simulink model "Sedimentation"  (R2024b)
settings: Solver=VariableStepAuto  StartTime=0.0  StopTime=1000  RelTol=1e-3
values from neighbouring files (symbols this model uses):
  b = Q_p/Q_in    (= 0.99)    [Input.m]
  D = Q_in/V    (= 0.166666666667)    [Input.m]
  f_ns = 1E-5    (= 1e-05)    [Input.m]
  h = 0.1    [Input.m]
  n = 5    [Input.m]
  r = Q_r/Q_in    (= 0.01)    [Input.m]
  r_h = 2E-6    (= 2e-06)    [Input.m]
  r_p = 1E-4    (= 0.0001)    [Input.m]
  v_0 = 10.42    [Input.m]
undefined symbols (not defined in the file or in its folder): X_in
settings Model: Creator=luima  LastModifiedBy=luima

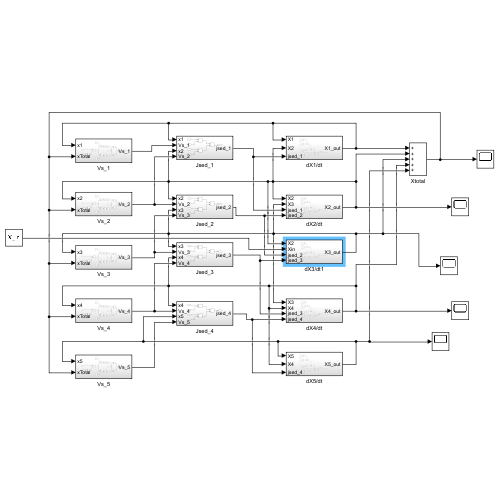
[thumbnail: Simulink's stored preview of the top-level diagram]
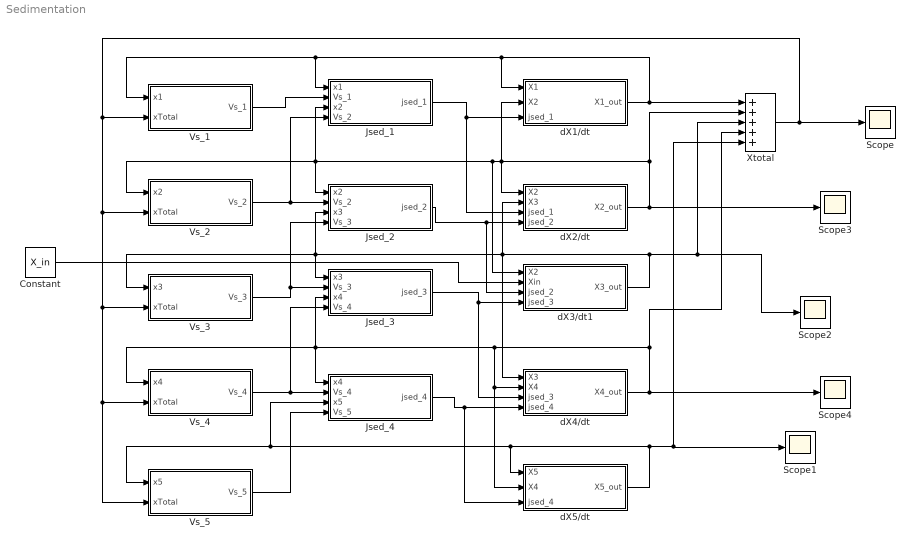
== system Sedimentation ==
  Constant : Constant  Value=X_in
  Jsed_1 : Subsystem
  Jsed_2 : Subsystem
  Jsed_3 : Subsystem
  Jsed_4 : Subsystem
  Scope{,1..4} (5 alike) : Scope
  Vs_1 : Subsystem
  Vs_2 : Subsystem
  Vs_3 : Subsystem
  Vs_4 : Subsystem
  Vs_5 : Subsystem
  Xtotal : Sum  Inputs=+++++
  dX1/dt : Subsystem
  dX2/dt : Subsystem
  dX3/dt1 : Subsystem
  dX4/dt : Subsystem
  dX5/dt : Subsystem
  wires:
  Vs_1/1(Vs_1) -> Jsed_1/2(Vs_1)
  Vs_2/1(Vs_2) -> Jsed_2/2(Vs_2), Jsed_1/4(Vs_2)
  Vs_3/1(Vs_3) -> Jsed_3/2(Vs_3), Jsed_2/4(Vs_3)
  Vs_4/1(Vs_4) -> Jsed_4/2(Vs_4), Jsed_3/4(Vs_4)
  Vs_5/1(Vs_5) -> Jsed_4/4(Vs_5)
  dX1/dt/1(X1_out) -> Xtotal/1, dX1/dt/1(X1), Jsed_1/1(x1), Vs_1/1(x1)
  dX2/dt/1(X2_out) -> Xtotal/2, Vs_2/1(x2), Jsed_1/3(x2), Jsed_2/1(x2), dX3/dt1/1(X2), dX1/dt/2(X2), dX2/dt/1(X2), Scope3/1
  Jsed_1/1(jsed_1) -> dX1/dt/3(jsed_1), dX2/dt/3(jsed_1)
  Jsed_2/1(jsed_2) -> dX3/dt1/3(jsed_2), dX2/dt/4(jsed_2)
  dX3/dt1/1(X3_out) -> Scope2/1, Xtotal/3, Vs_3/1(x3), Jsed_2/3(x3), Jsed_3/1(x3), dX4/dt/1(X3), dX2/dt/2(X3)
  Constant/1 -> dX3/dt1/2(Xin)
  Jsed_3/1(jsed_3) -> dX4/dt/3(jsed_3), dX3/dt1/4(jsed_3)
  dX4/dt/1(X4_out) -> Scope4/1, Xtotal/4, Vs_4/1(x4), Jsed_3/3(x4), Jsed_4/1(x4), dX4/dt/2(X4), dX5/dt/2(X4)
  Jsed_4/1(jsed_4) -> dX4/dt/4(jsed_4), dX5/dt/3(jsed_4)
  dX5/dt/1(X5_out) -> Xtotal/5, Scope1/1, Vs_5/1(x5), Jsed_4/3(x5), dX5/dt/1(X5)
  Xtotal/1 -> Scope/1, Vs_1/2(xTotal), Vs_3/2(xTotal), Vs_5/2(xTotal), Vs_4/2(xTotal), Vs_2/2(xTotal)

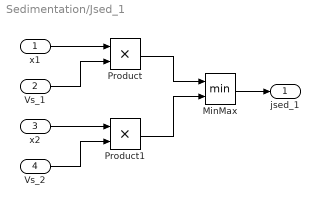
== system Sedimentation/Jsed_1 ==
  x1 : Inport
  Vs_1 : Inport  Port=2
  x2 : Inport  Port=3
  Vs_2 : Inport  Port=4
  MinMax : MinMax  Inputs=2
  Product : Product
  Product1 : Product
  jsed_1 : Outport
  wires:
  x1/1 -> Product/1
  Vs_1/1 -> Product/2
  x2/1 -> Product1/1
  Vs_2/1 -> Product1/2
  Product/1 -> MinMax/1
  Product1/1 -> MinMax/2
  MinMax/1 -> jsed_1/1

== system Sedimentation/Jsed_2 ==
  x2 : Inport
  Vs_2 : Inport  Port=2
  x3 : Inport  Port=3
  Vs_3 : Inport  Port=4
  MinMax : MinMax  Inputs=2
  Product : Product
  Product1 : Product
  jsed_2 : Outport
  wires:
  x2/1 -> Product/1
  Vs_2/1 -> Product/2
  x3/1 -> Product1/1
  Vs_3/1 -> Product1/2
  Product/1 -> MinMax/1
  Product1/1 -> MinMax/2
  MinMax/1 -> jsed_2/1

== system Sedimentation/Jsed_3 ==
  x3 : Inport
  Vs_3 : Inport  Port=2
  x4 : Inport  Port=3
  Vs_4 : Inport  Port=4
  MinMax : MinMax  Inputs=2
  Product : Product
  Product1 : Product
  jsed_3 : Outport
  wires:
  x3/1 -> Product/1
  Vs_3/1 -> Product/2
  x4/1 -> Product1/1
  Vs_4/1 -> Product1/2
  Product/1 -> MinMax/1
  Product1/1 -> MinMax/2
  MinMax/1 -> jsed_3/1

== system Sedimentation/Jsed_4 ==
  x4 : Inport
  Vs_4 : Inport  Port=2
  x5 : Inport  Port=3
  Vs_5 : Inport  Port=4
  MinMax : MinMax  Inputs=2
  Product : Product
  Product1 : Product
  jsed_4 : Outport
  wires:
  x4/1 -> Product/1
  Vs_4/1 -> Product/2
  x5/1 -> Product1/1
  Vs_5/1 -> Product1/2
  Product/1 -> MinMax/1
  Product1/1 -> MinMax/2
  MinMax/1 -> jsed_4/1

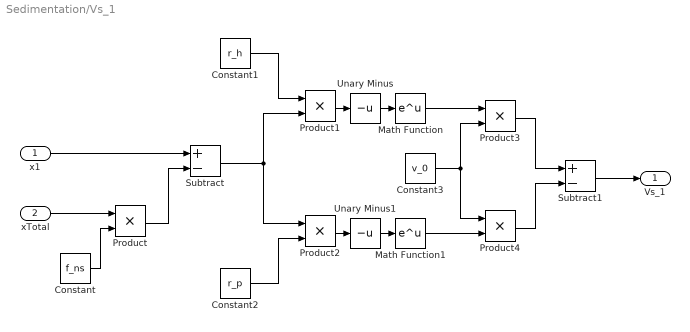
== system Sedimentation/Vs_1 ==
  x1 : Inport
  xTotal : Inport  Port=2
  Constant : Constant  Value=f_ns
  Constant1 : Constant  Value=r_h
  Constant2 : Constant  Value=r_p  VectorParams1D=off
  Constant3 : Constant  Value=v_0
  Math Function : Math
  Math Function1 : Math
  Product{,1..4} (5 alike) : Product
  Subtract : Sum  Inputs=+-
  Subtract1 : Sum  Inputs=+-
  Unary Minus : UnaryMinus
  Unary Minus1 : UnaryMinus
  Vs_1 : Outport
  wires:
  x1/1 -> Subtract/1
  xTotal/1 -> Product/1
  Constant/1 -> Product/2
  Product/1 -> Subtract/2
  Subtract/1 -> Product2/1, Product1/2
  Constant1/1 -> Product1/1
  Constant2/1 -> Product2/2
  Math Function/1 -> Product3/1
  Math Function1/1 -> Product4/2
  Constant3/1 -> Product3/2, Product4/1
  Product3/1 -> Subtract1/1
  Product4/1 -> Subtract1/2
  Subtract1/1 -> Vs_1/1
  Product1/1 -> Unary Minus/1
  Unary Minus/1 -> Math Function/1
  Product2/1 -> Unary Minus1/1
  Unary Minus1/1 -> Math Function1/1

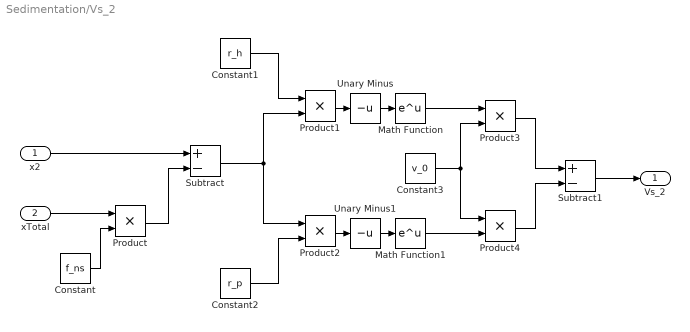
== system Sedimentation/Vs_2 ==
  x2 : Inport
  xTotal : Inport  Port=2
  Constant : Constant  Value=f_ns
  Constant1 : Constant  Value=r_h
  Constant2 : Constant  Value=r_p  VectorParams1D=off
  Constant3 : Constant  Value=v_0
  Math Function : Math
  Math Function1 : Math
  Product{,1..4} (5 alike) : Product
  Subtract : Sum  Inputs=+-
  Subtract1 : Sum  Inputs=+-
  Unary Minus : UnaryMinus
  Unary Minus1 : UnaryMinus
  Vs_2 : Outport
  wires:
  x2/1 -> Subtract/1
  xTotal/1 -> Product/1
  Constant/1 -> Product/2
  Product/1 -> Subtract/2
  Subtract/1 -> Product2/1, Product1/2
  Constant1/1 -> Product1/1
  Constant2/1 -> Product2/2
  Math Function/1 -> Product3/1
  Math Function1/1 -> Product4/2
  Constant3/1 -> Product3/2, Product4/1
  Product3/1 -> Subtract1/1
  Product4/1 -> Subtract1/2
  Subtract1/1 -> Vs_2/1
  Product1/1 -> Unary Minus/1
  Unary Minus/1 -> Math Function/1
  Product2/1 -> Unary Minus1/1
  Unary Minus1/1 -> Math Function1/1

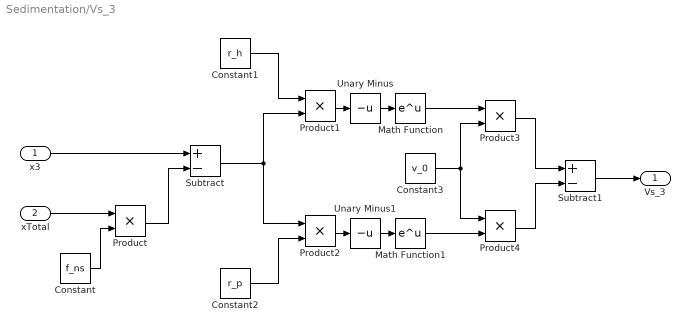
== system Sedimentation/Vs_3 ==
  x3 : Inport
  xTotal : Inport  Port=2
  Constant : Constant  Value=f_ns
  Constant1 : Constant  Value=r_h
  Constant2 : Constant  Value=r_p  VectorParams1D=off
  Constant3 : Constant  Value=v_0
  Math Function : Math
  Math Function1 : Math
  Product{,1..4} (5 alike) : Product
  Subtract : Sum  Inputs=+-
  Subtract1 : Sum  Inputs=+-
  Unary Minus : UnaryMinus
  Unary Minus1 : UnaryMinus
  Vs_3 : Outport
  wires:
  x3/1 -> Subtract/1
  xTotal/1 -> Product/1
  Constant/1 -> Product/2
  Product/1 -> Subtract/2
  Subtract/1 -> Product2/1, Product1/2
  Constant1/1 -> Product1/1
  Constant2/1 -> Product2/2
  Math Function/1 -> Product3/1
  Math Function1/1 -> Product4/2
  Constant3/1 -> Product3/2, Product4/1
  Product3/1 -> Subtract1/1
  Product4/1 -> Subtract1/2
  Subtract1/1 -> Vs_3/1
  Product1/1 -> Unary Minus/1
  Unary Minus/1 -> Math Function/1
  Product2/1 -> Unary Minus1/1
  Unary Minus1/1 -> Math Function1/1

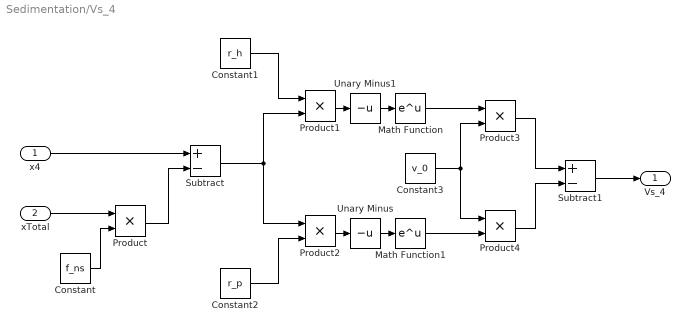
== system Sedimentation/Vs_4 ==
  x4 : Inport
  xTotal : Inport  Port=2
  Constant : Constant  Value=f_ns
  Constant1 : Constant  Value=r_h
  Constant2 : Constant  Value=r_p  VectorParams1D=off
  Constant3 : Constant  Value=v_0
  Math Function : Math
  Math Function1 : Math
  Product{,1..4} (5 alike) : Product
  Subtract : Sum  Inputs=+-
  Subtract1 : Sum  Inputs=+-
  Unary Minus : UnaryMinus
  Unary Minus1 : UnaryMinus
  Vs_4 : Outport
  wires:
  x4/1 -> Subtract/1
  xTotal/1 -> Product/1
  Constant/1 -> Product/2
  Product/1 -> Subtract/2
  Subtract/1 -> Product2/1, Product1/2
  Constant1/1 -> Product1/1
  Constant2/1 -> Product2/2
  Math Function/1 -> Product3/1
  Math Function1/1 -> Product4/2
  Constant3/1 -> Product3/2, Product4/1
  Product3/1 -> Subtract1/1
  Product4/1 -> Subtract1/2
  Subtract1/1 -> Vs_4/1
  Product1/1 -> Unary Minus1/1
  Unary Minus1/1 -> Math Function/1
  Product2/1 -> Unary Minus/1
  Unary Minus/1 -> Math Function1/1

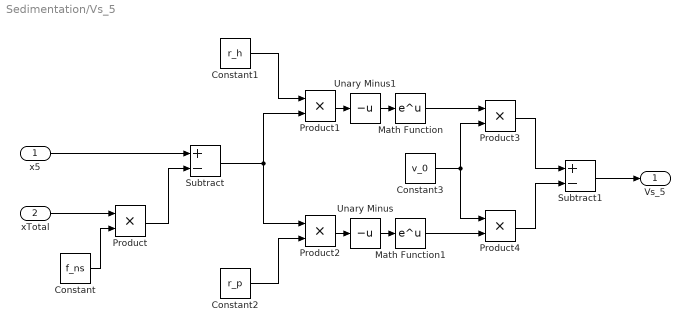
== system Sedimentation/Vs_5 ==
  x5 : Inport
  xTotal : Inport  Port=2
  Constant : Constant  Value=f_ns
  Constant1 : Constant  Value=r_h
  Constant2 : Constant  Value=r_p  VectorParams1D=off
  Constant3 : Constant  Value=v_0
  Math Function : Math
  Math Function1 : Math
  Product{,1..4} (5 alike) : Product
  Subtract : Sum  Inputs=+-
  Subtract1 : Sum  Inputs=+-
  Unary Minus : UnaryMinus
  Unary Minus1 : UnaryMinus
  Vs_5 : Outport
  wires:
  x5/1 -> Subtract/1
  xTotal/1 -> Product/1
  Constant/1 -> Product/2
  Product/1 -> Subtract/2
  Subtract/1 -> Product2/1, Product1/2
  Constant1/1 -> Product1/1
  Constant2/1 -> Product2/2
  Math Function/1 -> Product3/1
  Math Function1/1 -> Product4/2
  Constant3/1 -> Product3/2, Product4/1
  Product3/1 -> Subtract1/1
  Product4/1 -> Subtract1/2
  Subtract1/1 -> Vs_5/1
  Product1/1 -> Unary Minus1/1
  Unary Minus1/1 -> Math Function/1
  Product2/1 -> Unary Minus/1
  Unary Minus/1 -> Math Function1/1

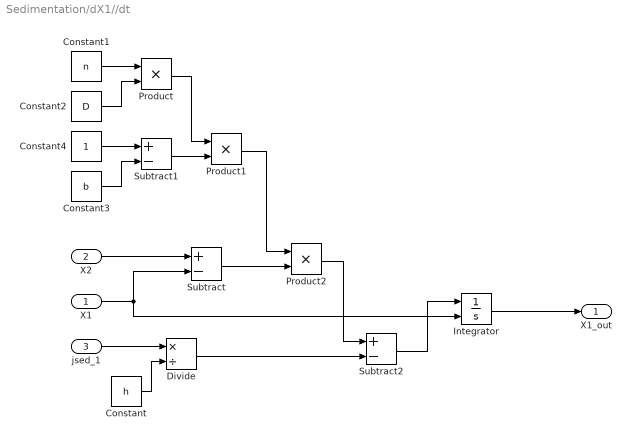
== system Sedimentation/dX1//dt ==
  X1 : Inport
  X2 : Inport  Port=2
  jsed_1 : Inport  Port=3
  Constant : Constant  Value=h
  Constant1 : Constant  Value=n
  Constant2 : Constant  Value=D
  Constant3 : Constant  Value=b
  Constant4 : Constant
  Divide : Product  Inputs=*/
  Integrator : Integrator  InitialConditionSource=external
  Product : Product
  Product1 : Product
  Product2 : Product
  Subtract : Sum  Inputs=+-
  Subtract1 : Sum  Inputs=+-
  Subtract2 : Sum  Inputs=+-
  X1_out : Outport
  wires:
  jsed_1/1 -> Divide/1
  Constant/1 -> Divide/2
  X2/1 -> Subtract/1
  X1/1 -> Integrator/2, Subtract/2
  Constant1/1 -> Product/1
  Constant2/1 -> Product/2
  Constant4/1 -> Subtract1/1
  Constant3/1 -> Subtract1/2
  Subtract1/1 -> Product1/2
  Product/1 -> Product1/1
  Subtract/1 -> Product2/2
  Product1/1 -> Product2/1
  Product2/1 -> Subtract2/1
  Divide/1 -> Subtract2/2
  Subtract2/1 -> Integrator/1
  Integrator/1 -> X1_out/1

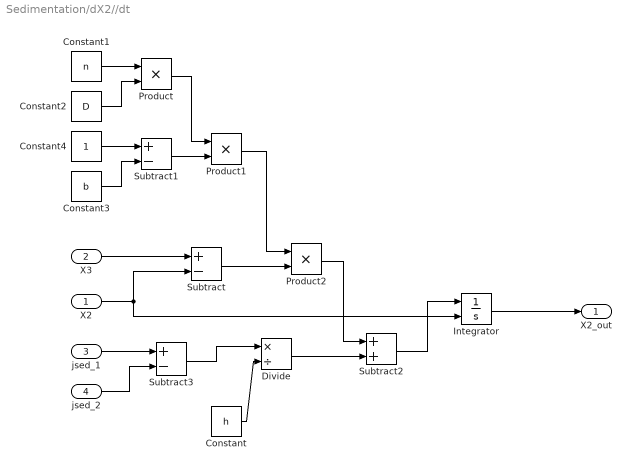
== system Sedimentation/dX2//dt ==
  X2 : Inport
  X3 : Inport  Port=2
  jsed_1 : Inport  Port=3
  jsed_2 : Inport  Port=4
  Constant : Constant  Value=h
  Constant1 : Constant  Value=n
  Constant2 : Constant  Value=D
  Constant3 : Constant  Value=b
  Constant4 : Constant
  Divide : Product  Inputs=*/
  Integrator : Integrator  InitialConditionSource=external
  Product : Product
  Product1 : Product
  Product2 : Product
  Subtract : Sum  Inputs=+-
  Subtract1 : Sum  Inputs=+-
  Subtract2 : Sum
  Subtract3 : Sum  Inputs=+-
  X2_out : Outport
  wires:
  Constant/1 -> Divide/2
  X3/1 -> Subtract/1
  X2/1 -> Integrator/2, Subtract/2
  Constant1/1 -> Product/1
  Constant2/1 -> Product/2
  Constant4/1 -> Subtract1/1
  Constant3/1 -> Subtract1/2
  Subtract1/1 -> Product1/2
  Product/1 -> Product1/1
  Subtract/1 -> Product2/2
  Product1/1 -> Product2/1
  Product2/1 -> Subtract2/1
  Divide/1 -> Subtract2/2
  Subtract2/1 -> Integrator/1
  Integrator/1 -> X2_out/1
  jsed_1/1 -> Subtract3/1
  jsed_2/1 -> Subtract3/2
  Subtract3/1 -> Divide/1

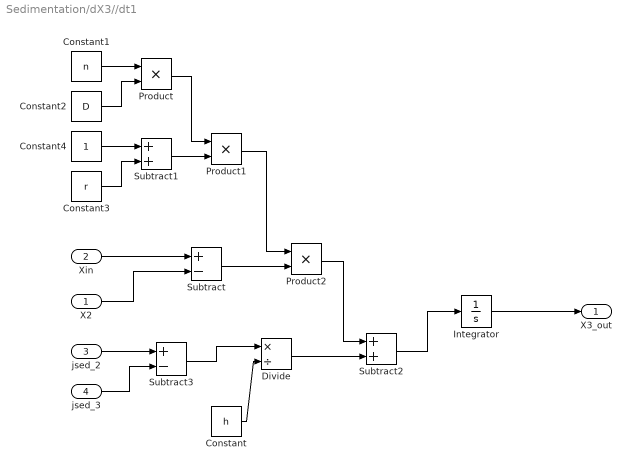
== system Sedimentation/dX3//dt1 ==
  X2 : Inport
  Xin : Inport  Port=2
  jsed_2 : Inport  Port=3
  jsed_3 : Inport  Port=4
  Constant : Constant  Value=h
  Constant1 : Constant  Value=n
  Constant2 : Constant  Value=D
  Constant3 : Constant  Value=r
  Constant4 : Constant
  Divide : Product  Inputs=*/
  Integrator : Integrator
  Product : Product
  Product1 : Product
  Product2 : Product
  Subtract : Sum  Inputs=+-
  Subtract1 : Sum
  Subtract2 : Sum
  Subtract3 : Sum  Inputs=+-
  X3_out : Outport
  wires:
  Constant/1 -> Divide/2
  Xin/1 -> Subtract/1
  X2/1 -> Subtract/2
  Constant1/1 -> Product/1
  Constant2/1 -> Product/2
  Constant4/1 -> Subtract1/1
  Constant3/1 -> Subtract1/2
  Subtract1/1 -> Product1/2
  Product/1 -> Product1/1
  Subtract/1 -> Product2/2
  Product1/1 -> Product2/1
  Product2/1 -> Subtract2/1
  Divide/1 -> Subtract2/2
  Subtract2/1 -> Integrator/1
  Integrator/1 -> X3_out/1
  jsed_2/1 -> Subtract3/1
  jsed_3/1 -> Subtract3/2
  Subtract3/1 -> Divide/1

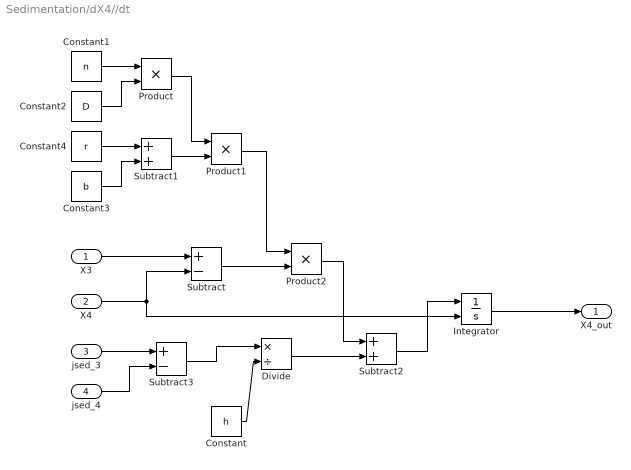
== system Sedimentation/dX4//dt ==
  X3 : Inport
  X4 : Inport  Port=2
  jsed_3 : Inport  Port=3
  jsed_4 : Inport  Port=4
  Constant : Constant  Value=h
  Constant1 : Constant  Value=n
  Constant2 : Constant  Value=D
  Constant3 : Constant  Value=b
  Constant4 : Constant  Value=r
  Divide : Product  Inputs=*/
  Integrator : Integrator  InitialConditionSource=external
  Product : Product
  Product1 : Product
  Product2 : Product
  Subtract : Sum  Inputs=+-
  Subtract1 : Sum
  Subtract2 : Sum
  Subtract3 : Sum  Inputs=+-
  X4_out : Outport
  wires:
  Constant/1 -> Divide/2
  Constant1/1 -> Product/1
  Constant2/1 -> Product/2
  Constant4/1 -> Subtract1/1
  Constant3/1 -> Subtract1/2
  Subtract1/1 -> Product1/2
  Product/1 -> Product1/1
  Subtract/1 -> Product2/2
  Product1/1 -> Product2/1
  Product2/1 -> Subtract2/1
  Divide/1 -> Subtract2/2
  Subtract2/1 -> Integrator/1
  Integrator/1 -> X4_out/1
  jsed_3/1 -> Subtract3/1
  jsed_4/1 -> Subtract3/2
  Subtract3/1 -> Divide/1
  X3/1 -> Subtract/1
  X4/1 -> Subtract/2, Integrator/2

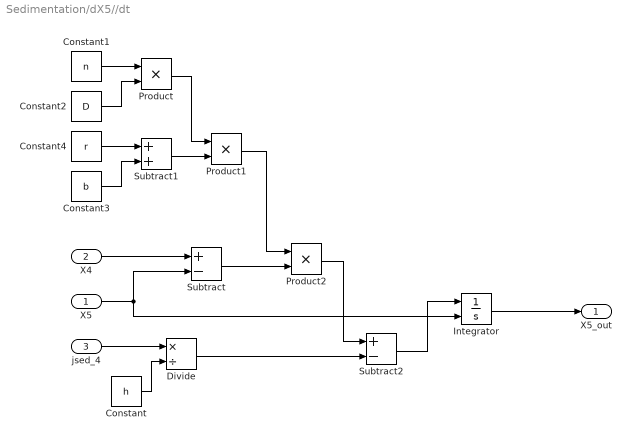
== system Sedimentation/dX5//dt ==
  X5 : Inport
  X4 : Inport  Port=2
  jsed_4 : Inport  Port=3
  Constant : Constant  Value=h
  Constant1 : Constant  Value=n
  Constant2 : Constant  Value=D
  Constant3 : Constant  Value=b
  Constant4 : Constant  Value=r
  Divide : Product  Inputs=*/
  Integrator : Integrator  InitialConditionSource=external
  Product : Product
  Product1 : Product
  Product2 : Product
  Subtract : Sum  Inputs=+-
  Subtract1 : Sum
  Subtract2 : Sum  Inputs=+-
  X5_out : Outport
  wires:
  jsed_4/1 -> Divide/1
  Constant/1 -> Divide/2
  X4/1 -> Subtract/1
  X5/1 -> Integrator/2, Subtract/2
  Constant1/1 -> Product/1
  Constant2/1 -> Product/2
  Constant4/1 -> Subtract1/1
  Constant3/1 -> Subtract1/2
  Subtract1/1 -> Product1/2
  Product/1 -> Product1/1
  Subtract/1 -> Product2/2
  Product1/1 -> Product2/1
  Product2/1 -> Subtract2/1
  Divide/1 -> Subtract2/2
  Subtract2/1 -> Integrator/1
  Integrator/1 -> X5_out/1
